simulink model "CylinderAdvancedOrbitModel"  (R2025b)
settings: Solver=ode4  StartTime=0.0  StopTime=20000  FixedStep=60  RelTol=1e-3
values from neighbouring files (symbols this model uses):
  Aref = 1.1666    [constantLoader.m]
  batCap = 300    [constantLoader.m]
  cd = 2.36    [constantLoader.m]
  eta = 0.6    [constantLoader.m]
  Isp = 3050    [constantLoader.m]
  SA_Area = P_S / (rho_EoL * cosd(SA_Theta))    [Power.m]    (also in constantLoader.m = 0.877)
  velocity = 7.7082 * 1000    (= 7708.2)    [constantLoader.m]
undefined symbols (not defined in the file or in its folder): IAU, juliandate
libraries: aerolibtransform2 x1, aerolibatmos2 x1
settings Model: Creator=mbgm9nc4  LastModifiedBy=ewanb

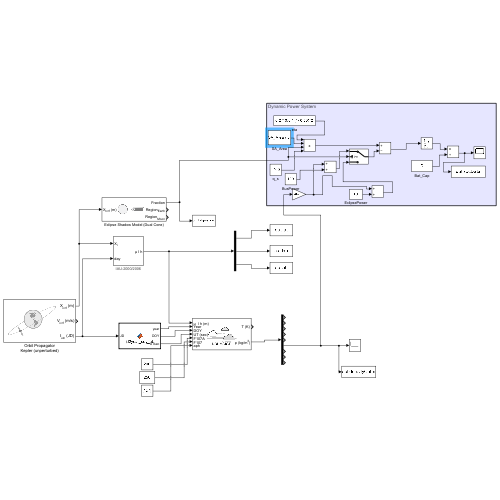
[thumbnail: Simulink's stored preview of the top-level diagram]
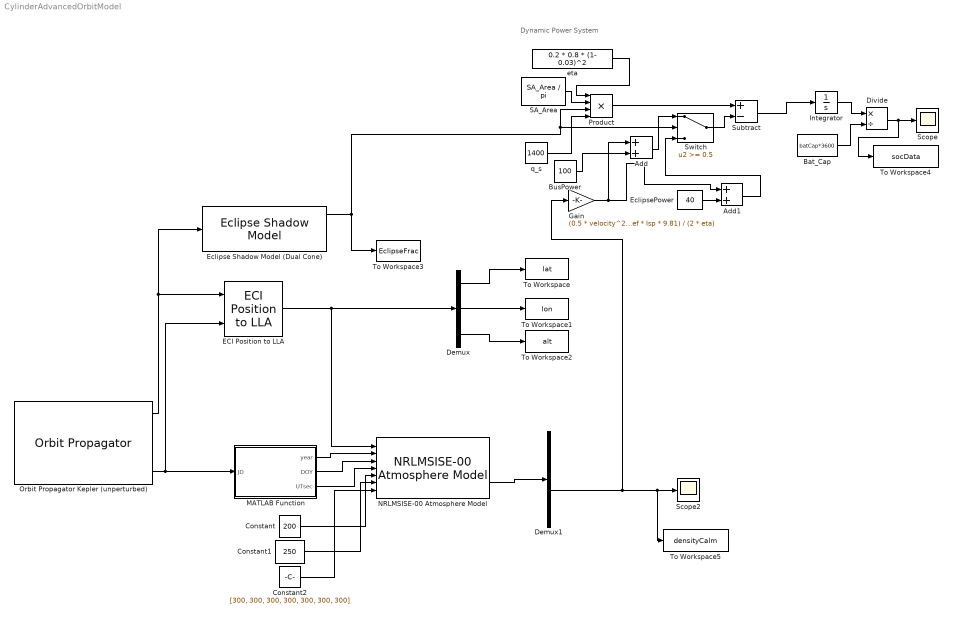
== system CylinderAdvancedOrbitModel ==
  note: Dynamic Power System
  Add : Sum
  Add1 : Sum
  Bat_Cap : Constant  Value=batCap*3600
  BusPower : Constant  Value=100
  Constant : Constant  Value=200
  Constant1 : Constant  Value=250
  Constant2 : Constant  Value=[300, 300, 300, 300, 300, 300, 300]
  Demux : Demux  Outputs=3
  Demux1 : Demux  Outputs=9
  Divide : Product  Inputs=*/
  ECI Position to LLA : aerolibtransform2/ECI Position to LLA  red=IAU-2000/2006  year=2013  month=January  day=1  hour=0  min=0  sec=0  deltaT=Day  errorflag=Error  extraparamflag=off  eunits=Metric (MKS)  earthmodel=WGS84  flat=1/298.257223563  eqradius=6378137
      settings: AttributesFormatString=%<red>
  Eclipse Shadow Model (Dual Cone) : EclipseShadowModel  shadowModel=Cylindrical  outputShadowRegion=on
  EclipsePower : Constant  Value=40
  Gain : Gain  Gain=(0.5 * velocity^2 * cd * Aref * Isp * 9.81) / (2 * eta)
  Integrator : Integrator  InitialCondition=batCap*3600  LimitOutput=on  UpperSaturationLimit=batCap * 3600  LowerSaturationLimit=0
  MATLAB Function : MATLAB Function  TreatAsAtomicUnit=on
  NRLMSISE-00 Atmosphere Model : aerolibatmos2/NRLMSISE-00 Atmosphere Model  units=Metric (MKS)  lst_input=off  flux_ap_input=on  flags_input=Internal  flags=ones(1,23)  oxygen_in=off  action=Warning
  Orbit Propagator Kepler (unperturbed) : OrbitPropagator  startDate=juliandate(2026, 3, 20, 12, 0, 0)  semiMajorAxis=(6378+330.5)*1000  eccentricity=0  inclination=96.78  raan=337.5  argPeriapsis=0  trueAnomaly=0  inertialPosition=[3649700.0 3308200.0 -4676600.0]  inertialVelocity=[-2750.8 6666.4 2573.4]  fixedPosition=[-4142689.0 -2676864.7 -4669861.6]  fixedVelocity=[1452.7 -6720.7 2568.1]  customR=3396200  customMu=4.305e13  customJ2=1.0826269e-03  customOmega=4.06125949e-3
  Product : Product  Inputs=4
  SA_Area : Constant  Value=SA_Area / pi
  Scope : Scope
      settings: ActiveDisplayYMinimum=-0.58183440779023132  ActiveDisplayYMaximum=1.7487655039531176
  Scope2 : Scope
      settings: ActiveDisplayYMinimum=2.6737241024671831E-11  ActiveDisplayYMaximum=6.49512301737929E-11
  Subtract : Sum  Inputs=+-
  Switch : Switch  Threshold=0.5  SaturateOnIntegerOverflow=off  InputSameDT=off
  To Workspace : ToWorkspace  VariableName=lat  SaveFormat=Timeseries  SampleTime=-1
  To Workspace1 : ToWorkspace  VariableName=lon  SaveFormat=Timeseries  SampleTime=-1
  To Workspace2 : ToWorkspace  VariableName=alt  SaveFormat=Timeseries  SampleTime=-1
  To Workspace3 : ToWorkspace  VariableName=EclipseFrac  SaveFormat=Timeseries  SampleTime=-1
  To Workspace4 : ToWorkspace  VariableName=socData  SampleTime=-1
  To Workspace5 : ToWorkspace  VariableName=densityCalm  SampleTime=-1
      settings: Save2DSignal=2-D array (concatenate along first dimension)
  eta : Constant  Value=0.2 * 0.8 * (1- 0.03)^2
  q_s : Constant  Value=1400
  wires:
  Demux/2 -> To Workspace1/1
  q_s/1 -> Product/4
  Bat_Cap/1 -> Divide/2
  Subtract/1 -> Integrator/1
  Demux/3 -> To Workspace2/1
  eta/1 -> Product/1
  SA_Area/1 -> Product/2
  Orbit Propagator Kepler (unperturbed)/1 -> Eclipse Shadow Model (Dual Cone)/1, ECI Position to LLA/1
  Product/1 -> Subtract/1
  MATLAB Function/2(DOY) -> NRLMSISE-00 Atmosphere Model/3
  Integrator/1 -> Divide/1
  ECI Position to LLA/1 -> NRLMSISE-00 Atmosphere Model/1, Demux/1
  Divide/1 -> To Workspace4/1, Scope/1
  Orbit Propagator Kepler (unperturbed)/3 -> ECI Position to LLA/2, MATLAB Function/1(JD)
  MATLAB Function/1(year) -> NRLMSISE-00 Atmosphere Model/2
  MATLAB Function/3(UTsec) -> NRLMSISE-00 Atmosphere Model/4
  Demux/1 -> To Workspace/1
  NRLMSISE-00 Atmosphere Model/2 -> Demux1/1
  Eclipse Shadow Model (Dual Cone)/1 -> Product/3, Switch/2, To Workspace3/1
  Switch/1 -> Subtract/2
  Add/1 -> Switch/1
  Add1/1 -> Switch/3
  Constant/1 -> NRLMSISE-00 Atmosphere Model/5
  Constant1/1 -> NRLMSISE-00 Atmosphere Model/6
  Constant2/1 -> NRLMSISE-00 Atmosphere Model/7
  Demux1/6 -> Gain/1, Scope2/1, To Workspace5/1
  Gain/1 -> Add/1, Add1/1
  BusPower/1 -> Add/2
  EclipsePower/1 -> Add1/2

== matlab function CylinderAdvancedOrbitModel/MATLAB Function ==
  data: year output; JD input; DOY output; UTsec output
function [year, DOY, UTsec] = jd2year_doy_ut(JD)
% Input:
%   JD   - Julian Date (UTC)
% Outputs:
%   year  - Gregorian year
%   DOY   - Day of year (1–366)
%   UTsec - Seconds past 00:00:00 UTC

% ---- Shift because JD starts at noon
JD_shift = JD + 0.5;
Z = floor(JD_shift);
F = JD_shift - Z;

% ---- UT seconds
UTsec = F * 86400.0;

% ---- Gregorian calendar conversion (Fliegel–Van Flandern)
alpha = floor((Z - 1867216.25)/36524.25);
A = Z + 1 + alpha - floor(alpha/4);
B = A + 1524;
C = floor((B - 122.1)/365.25);
D = floor(365.25 * C);
E = floor((B - D)/30.6001);
day = B - D - floor(30.6001 * E);

if E < 14
    month = E - 1;
else
    month = E - 13;
end

if month > 2
    year = C - 4716;
else
    year = C - 4715;
end

% ---- Compute DOY
% Leap year test
isLeap = (mod(year,4)==0 && mod(year,100)~=0) || mod(year,400)==0;
monthDays = [31 28+isLeap 31 30 31 30 31 31 30 31 30 31];
DOY = day;
for k = 1:month-1
    DOY = DOY + monthDays(k);
end

end
